simulink model "PS1_sim"  (R2017a)
settings: Solver=VariableStepAuto  StartTime=0.0  StopTime=5  RelTol=1e-3
values from neighbouring files (symbols this model uses):
  den = [Rf*C, 1]    [HW2_P2_Mat.m]    (also in PS1.m = [1/(2000^2), 2.0000e-05, 1]; PS1_1.m = [1 30 100])
  e_i = 5    [PS1_1.m]
  num = (-Rf/Ri)    (= -100)    [HW2_P2_Mat.m]    (also in PS1.m = 1; PS1_1.m = 100)
settings Model: Creator=Shaun  LastModifiedBy=Shaun

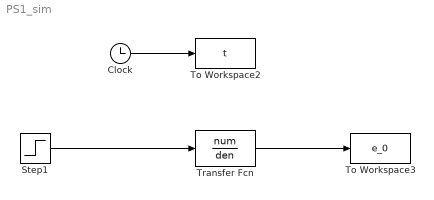
== system PS1_sim ==
  Clock : Clock
  Step1 : Step  Time=.5  After=e_i  SampleTime=0
  To Workspace2 : ToWorkspace  VariableName=t  SampleTime=-1
  To Workspace3 : ToWorkspace  VariableName=e_0  SampleTime=-1
  Transfer Fcn : TransferFcn  Numerator=num  Denominator=den
  wires:
  Clock/1 -> To Workspace2/1
  Step1/1 -> Transfer Fcn/1
  Transfer Fcn/1 -> To Workspace3/1
